simulink library "CryoDetLibCMB"  (R2016b)
settings: Solver=VariableStepAuto  StartTime=0.0  StopTime=10.0  RelTol=1e-3
undefined symbols (not defined in the file): Fclk, xlipgetpartsetting
libraries: xbsIndex_r4 x329, CryoDetLibCMB x20, CryoDetLib x2, simulink x1
(part 2 of 3)

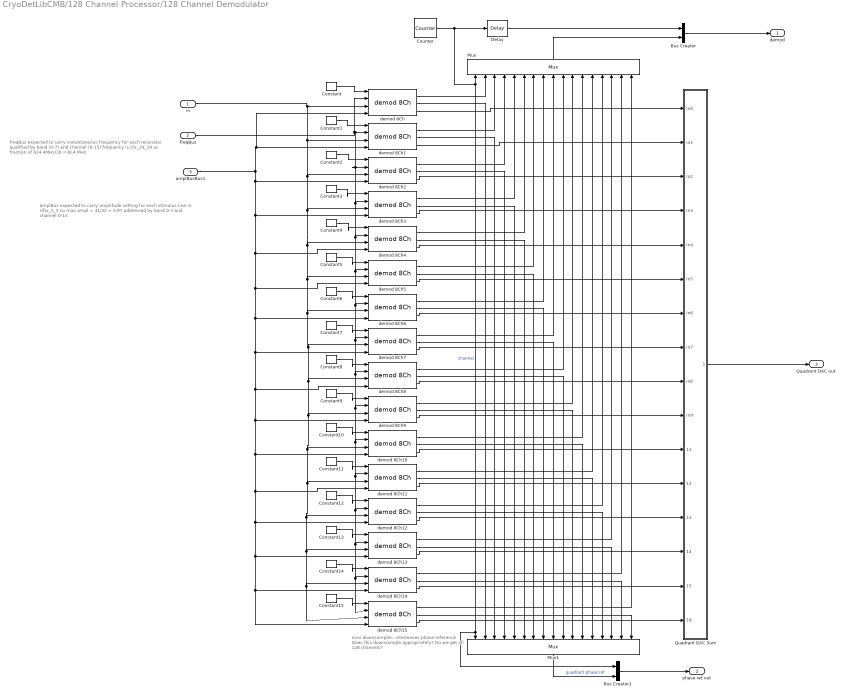
== system CryoDetLibCMB/128 Channel Processor/128 Channel Demodulator ==
  note: amplBus expected to carry  amplitude setting for each stimulus line
      | in Ufix_5_5 so max ampl = 31/32 = 0.97
      | addressed by band 0-7 and channel 0-15
  note: freqBus expected to carry instantaneous frequency for each resonator
      | qualified by band (0-7) and channel (0-15)
      | frequency is Fix_24_24 as fraction of 614.4MHz/16 =38.4 MHz
  note: mux downsamples, interleaves phase reference
      | Does this downsample appropriately?
      | Do we get all 128 channels?
  in : Inport
  freqBus : Inport  Port=2
  amplBusBus1 : Inport  Port=3
  Bus Creator : BusCreator  Inputs=2
  Bus Creator1 : BusCreator  Inputs=2
  Constant : xbsIndex_r4/Constant  const=0  gui_display_data_type=Fixed-point  arith_type=Unsigned  n_bits=4  bin_pt=0  preci_type=Single  exp_width=8  frac_width=24  explicit_period=off  period=1  equ=P=C  opselect=C  inp2=PCIN>>17  opr=+  inp1=P  carry=CIN  dbl_ovrd=off  block_type=constant
  Constant1 : xbsIndex_r4/Constant  const=1  gui_display_data_type=Fixed-point  arith_type=Unsigned  n_bits=4  bin_pt=0  preci_type=Single  exp_width=8  frac_width=24  explicit_period=off  period=1  equ=P=C  opselect=C  inp2=PCIN>>17  opr=+  inp1=P  carry=CIN  dbl_ovrd=off  block_type=constant
  Constant10 : xbsIndex_r4/Constant  const=10  gui_display_data_type=Fixed-point  arith_type=Unsigned  n_bits=4  bin_pt=0  preci_type=Single  exp_width=8  frac_width=24  explicit_period=off  period=1  equ=P=C  opselect=C  inp2=PCIN>>17  opr=+  inp1=P  carry=CIN  dbl_ovrd=off  block_type=constant
  Constant11 : xbsIndex_r4/Constant  const=11  gui_display_data_type=Fixed-point  arith_type=Unsigned  n_bits=4  bin_pt=0  preci_type=Single  exp_width=8  frac_width=24  explicit_period=off  period=1  equ=P=C  opselect=C  inp2=PCIN>>17  opr=+  inp1=P  carry=CIN  dbl_ovrd=off  block_type=constant
  Constant12 : xbsIndex_r4/Constant  const=12  gui_display_data_type=Fixed-point  arith_type=Unsigned  n_bits=4  bin_pt=0  preci_type=Single  exp_width=8  frac_width=24  explicit_period=off  period=1  equ=P=C  opselect=C  inp2=PCIN>>17  opr=+  inp1=P  carry=CIN  dbl_ovrd=off  block_type=constant
  Constant13 : xbsIndex_r4/Constant  const=13  gui_display_data_type=Fixed-point  arith_type=Unsigned  n_bits=4  bin_pt=0  preci_type=Single  exp_width=8  frac_width=24  explicit_period=off  period=1  equ=P=C  opselect=C  inp2=PCIN>>17  opr=+  inp1=P  carry=CIN  dbl_ovrd=off  block_type=constant
  Constant14 : xbsIndex_r4/Constant  const=14  gui_display_data_type=Fixed-point  arith_type=Unsigned  n_bits=4  bin_pt=0  preci_type=Single  exp_width=8  frac_width=24  explicit_period=off  period=1  equ=P=C  opselect=C  inp2=PCIN>>17  opr=+  inp1=P  carry=CIN  dbl_ovrd=off  block_type=constant
  Constant15 : xbsIndex_r4/Constant  const=15  gui_display_data_type=Fixed-point  arith_type=Unsigned  n_bits=4  bin_pt=0  preci_type=Single  exp_width=8  frac_width=24  explicit_period=off  period=1  equ=P=C  opselect=C  inp2=PCIN>>17  opr=+  inp1=P  carry=CIN  dbl_ovrd=off  block_type=constant
  Constant2 : xbsIndex_r4/Constant  const=2  gui_display_data_type=Fixed-point  arith_type=Unsigned  n_bits=4  bin_pt=0  preci_type=Single  exp_width=8  frac_width=24  explicit_period=off  period=1  equ=P=C  opselect=C  inp2=PCIN>>17  opr=+  inp1=P  carry=CIN  dbl_ovrd=off  block_type=constant
  Constant3 : xbsIndex_r4/Constant  const=3  gui_display_data_type=Fixed-point  arith_type=Unsigned  n_bits=4  bin_pt=0  preci_type=Single  exp_width=8  frac_width=24  explicit_period=off  period=1  equ=P=C  opselect=C  inp2=PCIN>>17  opr=+  inp1=P  carry=CIN  dbl_ovrd=off  block_type=constant
  Constant4 : xbsIndex_r4/Constant  const=4  gui_display_data_type=Fixed-point  arith_type=Unsigned  n_bits=4  bin_pt=0  preci_type=Single  exp_width=8  frac_width=24  explicit_period=off  period=1  equ=P=C  opselect=C  inp2=PCIN>>17  opr=+  inp1=P  carry=CIN  dbl_ovrd=off  block_type=constant
  Constant5 : xbsIndex_r4/Constant  const=5  gui_display_data_type=Fixed-point  arith_type=Unsigned  n_bits=4  bin_pt=0  preci_type=Single  exp_width=8  frac_width=24  explicit_period=off  period=1  equ=P=C  opselect=C  inp2=PCIN>>17  opr=+  inp1=P  carry=CIN  dbl_ovrd=off  block_type=constant
  Constant6 : xbsIndex_r4/Constant  const=6  gui_display_data_type=Fixed-point  arith_type=Unsigned  n_bits=4  bin_pt=0  preci_type=Single  exp_width=8  frac_width=24  explicit_period=off  period=1  equ=P=C  opselect=C  inp2=PCIN>>17  opr=+  inp1=P  carry=CIN  dbl_ovrd=off  block_type=constant
  Constant7 : xbsIndex_r4/Constant  const=7  gui_display_data_type=Fixed-point  arith_type=Unsigned  n_bits=4  bin_pt=0  preci_type=Single  exp_width=8  frac_width=24  explicit_period=off  period=1  equ=P=C  opselect=C  inp2=PCIN>>17  opr=+  inp1=P  carry=CIN  dbl_ovrd=off  block_type=constant
  Constant8 : xbsIndex_r4/Constant  const=8  gui_display_data_type=Fixed-point  arith_type=Unsigned  n_bits=4  bin_pt=0  preci_type=Single  exp_width=8  frac_width=24  explicit_period=off  period=1  equ=P=C  opselect=C  inp2=PCIN>>17  opr=+  inp1=P  carry=CIN  dbl_ovrd=off  block_type=constant
  Constant9 : xbsIndex_r4/Constant  const=9  gui_display_data_type=Fixed-point  arith_type=Unsigned  n_bits=4  bin_pt=0  preci_type=Single  exp_width=8  frac_width=24  explicit_period=off  period=1  equ=P=C  opselect=C  inp2=PCIN>>17  opr=+  inp1=P  carry=CIN  dbl_ovrd=off  block_type=constant
  Counter : xbsIndex_r4/Counter  cnt_type=Free Running  cnt_to=Inf  operation=Up  start_count=0  cnt_by_val=1  arith_type=Unsigned  n_bits=4  bin_pt=0  load_pin=off  rst=off  en=off  explicit_period=on  period=Tclk  use_behavioral_HDL=off  implementation=Fabric  dbl_ovrd=off  block_type=counter
  Delay : xbsIndex_r4/Delay  rst=off  infoeditControl=Selection of Reset will increase slice count due to use of real FFs and instead of SRLs  en=off  latency=1  reg_retiming=off  dbl_ovrd=off  block_type=delay
  Mux : xbsIndex_r4/Mux  inputs=16  en=off  latency=1  precision=Full  arith_type=Unsigned  n_bits=16  bin_pt=14  quantization=Truncate  overflow=Wrap  dbl_ovrd=off  block_type=mux
  Mux1 : xbsIndex_r4/Mux  inputs=16  en=off  latency=1  precision=Full  arith_type=Unsigned  n_bits=16  bin_pt=14  quantization=Truncate  overflow=Wrap  dbl_ovrd=off  block_type=mux
  Quadrant DAC Sum : Subsystem
  demod 8Ch{,1..15} (16 alike) : CryoDetLibCMB/demod 8Ch
  demod : Outport
  phase ref out : Outport  Port=2
  Quadrant DAC out : Outport  Port=3
  wires:
  Constant/1 -> demod 8Ch/1
  Constant1/1 -> demod 8Ch1/1
  Constant2/1 -> demod 8Ch2/1
  Constant3/1 -> demod 8Ch3/1
  Constant4/1 -> demod 8Ch4/1
  Constant5/1 -> demod 8Ch5/1
  Constant6/1 -> demod 8Ch6/1
  Constant7/1 -> demod 8Ch7/1
  Constant8/1 -> demod 8Ch8/1
  Constant9/1 -> demod 8Ch9/1
  Constant10/1 -> demod 8Ch10/1
  Constant11/1 -> demod 8Ch11/1
  Constant12/1 -> demod 8Ch12/1
  Constant13/1 -> demod 8Ch13/1
  Constant14/1 -> demod 8Ch14/1
  freqBus/1 -> demod 8Ch2/2, demod 8Ch5/2, demod 8Ch6/2, demod 8Ch7/2, demod 8Ch8/2, demod 8Ch10/2, demod 8Ch11/2, demod 8Ch12/2, demod 8Ch13/2, demod 8Ch14/2, demod 8Ch15/2, demod 8Ch9/2, demod 8Ch4/2, demod 8Ch3/2, demod 8Ch1/2, demod 8Ch/2
  demod 8Ch/1 -> Mux/2
  Counter/1 -> Delay/1, Bus Creator1/1, Mux1/1, Mux/1  "channel"
  Delay/1 -> Bus Creator/1
  Mux/1 -> Bus Creator/2
  demod 8Ch1/1 -> Mux/3
  demod 8Ch2/1 -> Mux/4
  demod 8Ch3/1 -> Mux/5
  demod 8Ch4/1 -> Mux/6
  demod 8Ch5/1 -> Mux/7
  demod 8Ch/2 -> Mux1/2
  demod 8Ch1/2 -> Mux1/3
  demod 8Ch2/2 -> Mux1/4
  demod 8Ch3/2 -> Mux1/5
  demod 8Ch4/2 -> Mux1/6
  demod 8Ch5/2 -> Mux1/7
  demod 8Ch/3 -> Quadrant DAC Sum/1(In0)
  demod 8Ch1/3 -> Quadrant DAC Sum/2(In1)
  demod 8Ch2/3 -> Quadrant DAC Sum/3(In2)
  demod 8Ch3/3 -> Quadrant DAC Sum/4(In3)
  demod 8Ch4/3 -> Quadrant DAC Sum/5(In4)
  demod 8Ch5/3 -> Quadrant DAC Sum/6(In5)
  demod 8Ch6/3 -> Quadrant DAC Sum/7(In6)
  demod 8Ch7/3 -> Quadrant DAC Sum/8(In7)
  demod 8Ch8/3 -> Quadrant DAC Sum/9(In8)
  demod 8Ch9/3 -> Quadrant DAC Sum/10(In9)
  demod 8Ch10/3 -> Quadrant DAC Sum/11(In10)
  demod 8Ch11/3 -> Quadrant DAC Sum/12(In11)
  demod 8Ch12/3 -> Quadrant DAC Sum/13(In12)
  demod 8Ch13/3 -> Quadrant DAC Sum/14(In13)
  demod 8Ch14/3 -> Quadrant DAC Sum/15(In14)
  Constant15/1 -> demod 8Ch15/1
  demod 8Ch15/3 -> Quadrant DAC Sum/16(In15)
  demod 8Ch15/2 -> Mux1/17
  demod 8Ch14/2 -> Mux1/16
  demod 8Ch13/2 -> Mux1/15
  demod 8Ch6/1 -> Mux/8
  demod 8Ch7/1 -> Mux/9
  demod 8Ch8/1 -> Mux/10
  demod 8Ch9/1 -> Mux/11
  demod 8Ch10/1 -> Mux/12
  demod 8Ch11/1 -> Mux/13
  demod 8Ch12/1 -> Mux/14
  demod 8Ch13/1 -> Mux/15
  demod 8Ch14/1 -> Mux/16
  demod 8Ch15/1 -> Mux/17
  demod 8Ch6/2 -> Mux1/8
  demod 8Ch12/2 -> Mux1/14
  demod 8Ch11/2 -> Mux1/13
  demod 8Ch10/2 -> Mux1/12
  demod 8Ch9/2 -> Mux1/11
  demod 8Ch7/2 -> Mux1/9
  demod 8Ch8/2 -> Mux1/10
  Mux1/1 -> Bus Creator1/2  "quadrant phase ref"
  Bus Creator1/1 -> phase ref out/1
  in/1 -> demod 8Ch/3, demod 8Ch2/3, demod 8Ch6/3, demod 8Ch7/3, demod 8Ch8/3, demod 8Ch10/3, demod 8Ch12/3, demod 8Ch15/3, demod 8Ch14/3, demod 8Ch13/3, demod 8Ch11/3, demod 8Ch9/3, demod 8Ch5/3, demod 8Ch4/3, demod 8Ch3/3, demod 8Ch1/3
  Bus Creator/1 -> demod/1
  Quadrant DAC Sum/1(Out2) -> Quadrant DAC out/1
  amplBusBus1/1 -> demod 8Ch/4, demod 8Ch1/4, demod 8Ch4/4, demod 8Ch5/4, demod 8Ch6/4, demod 8Ch7/4, demod 8Ch8/4, demod 8Ch9/4, demod 8Ch10/4, demod 8Ch11/4, demod 8Ch12/4, demod 8Ch13/4, demod 8Ch14/4, demod 8Ch15/4, demod 8Ch3/4, demod 8Ch2/4

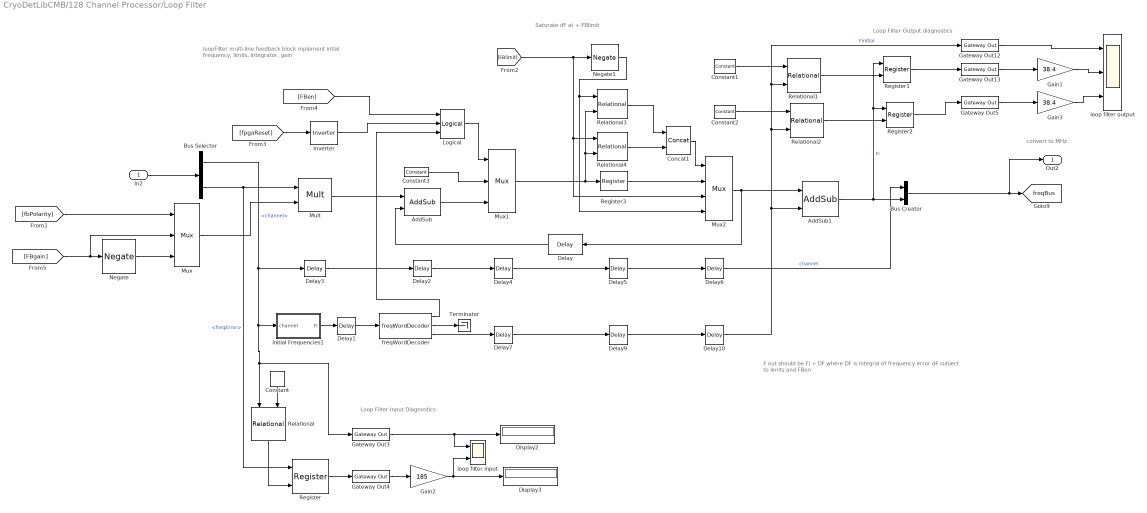
== system CryoDetLibCMB/128 Channel Processor/Loop Filter ==
  note: Loop Filter Output diagnostics
  note: Loop Filter Input Diagnostics
  note: Saturate dF at +-FBlimit
  note: convert to MHz
  note: F out should be Fi + DF
      | where DF is integral of frequency error dF subject to limits and FBen
  note: loopFilter
      | multi-line feedback block
      | mplement intial frequency, limits, integrator, gain
  In2 : Inport
  AddSub : xbsIndex_r4/AddSub  mode=Addition  use_carryin=off  use_carryout=off  en=off  latency=1  precision=User Defined  arith_type="Signed  (2's comp)"  n_bits=32  bin_pt=30  quantization=Truncate  overflow=Saturate  use_behavioral_HDL=off  hw_selection=Fabric  pipelined=off  dbl_ovrd=off  block_type=addsub
  AddSub1 : xbsIndex_r4/AddSub  mode=Addition  use_carryin=off  use_carryout=off  en=off  latency=1  precision=Full  arith_type=Unsigned  n_bits=16  bin_pt=14  quantization=Truncate  overflow=Wrap  use_behavioral_HDL=off  hw_selection=Fabric  pipelined=off  dbl_ovrd=off  block_type=addsub
  Bus Selector : BusSelector  OutputSignals=channel,freqError
  Bus Creator : BusCreator  Inputs=2
  Concat1 : xbsIndex_r4/Concat  num_inputs=2  dbl_ovrd=off  block_type=concat
  Constant : xbsIndex_r4/Constant  const=0  gui_display_data_type=Fixed-point  arith_type=Unsigned  n_bits=4  bin_pt=0  preci_type=Single  exp_width=8  frac_width=24  explicit_period=off  period=1  equ=P=C  opselect=C  inp2=PCIN>>17  opr=+  inp1=P  carry=CIN  dbl_ovrd=off  block_type=constant
  Constant1 : xbsIndex_r4/Constant  const=0  gui_display_data_type=Fixed-point  arith_type=Unsigned  n_bits=4  bin_pt=0  preci_type=Single  exp_width=8  frac_width=24  explicit_period=off  period=1  equ=P=C  opselect=C  inp2=PCIN>>17  opr=+  inp1=P  carry=CIN  dbl_ovrd=off  block_type=constant
  Constant2 : xbsIndex_r4/Constant  const=6  gui_display_data_type=Fixed-point  arith_type=Unsigned  n_bits=4  bin_pt=0  preci_type=Single  exp_width=8  frac_width=24  explicit_period=off  period=1  equ=P=C  opselect=C  inp2=PCIN>>17  opr=+  inp1=P  carry=CIN  dbl_ovrd=off  block_type=constant
  Constant3 : xbsIndex_r4/Constant  const=0  gui_display_data_type=Fixed-point  arith_type=Signed (2's comp)  n_bits=32  bin_pt=30  preci_type=Single  exp_width=8  frac_width=24  explicit_period=off  period=1  equ=P=C  opselect=C  inp2=PCIN>>17  opr=+  inp1=P  carry=CIN  dbl_ovrd=off  block_type=constant
  Delay : xbsIndex_r4/Delay  rst=off  infoeditControl=Selection of Reset will increase slice count due to use of real FFs and instead of SRLs  en=off  latency=124  reg_retiming=off  dbl_ovrd=off  block_type=delay
  Delay1 : xbsIndex_r4/Delay  rst=off  infoeditControl=Selection of Reset will increase slice count due to use of real FFs and instead of SRLs  en=off  latency=2  reg_retiming=off  dbl_ovrd=off  block_type=delay
  Delay{2,4..6,9..10} (6 alike) : xbsIndex_r4/Delay  rst=off  infoeditControl=Selection of Reset will increase slice count due to use of real FFs and instead of SRLs  en=off  latency=1  reg_retiming=off  dbl_ovrd=off  block_type=delay
  Delay3 : xbsIndex_r4/Delay  rst=off  infoeditControl=Selection of Reset will increase slice count due to use of real FFs and instead of SRLs  en=off  latency=3  reg_retiming=off  dbl_ovrd=off  block_type=delay
  Delay7 : xbsIndex_r4/Delay  rst=off  infoeditControl=Selection of Reset will increase slice count due to use of real FFs and instead of SRLs  en=off  latency=2  reg_retiming=off  dbl_ovrd=off  block_type=delay
  Display2 : Display
  Display3 : Display
  Gain1 : Gain  Gain=38.4
  Gain2 : Gain  Gain=185
  Gain3 : Gain  Gain=38.4
  Gateway Out12 : xbsIndex_r4/Gateway Out  inherit_from_input=off  hdl_port=off  rows=1  columns=1  UseAsDAC=off  DACChannel='1'  interface=None  automatic_assignment=on  address_offset=hex2dec('00')  intf_name=''  intf_description=''  timing_constraint=None  locs_specified=off  LOCs={}  io_standard={}  block_type=gatewayout
  Gateway Out13 : xbsIndex_r4/Gateway Out  inherit_from_input=on  hdl_port=off  rows=1  columns=1  UseAsDAC=off  DACChannel='1'  interface=None  automatic_assignment=on  address_offset=hex2dec('00')  intf_name=''  intf_description=''  timing_constraint=None  locs_specified=off  LOCs={}  io_standard={}  block_type=gatewayout
  Gateway Out3 : xbsIndex_r4/Gateway Out  inherit_from_input=off  hdl_port=off  rows=1  columns=1  UseAsDAC=off  DACChannel='1'  interface=None  automatic_assignment=on  address_offset=hex2dec('00')  intf_name=''  intf_description=''  timing_constraint=None  locs_specified=off  LOCs={}  io_standard={}  block_type=gatewayout
  Gateway Out4 : xbsIndex_r4/Gateway Out  inherit_from_input=off  hdl_port=off  rows=1  columns=1  UseAsDAC=off  DACChannel='1'  interface=None  automatic_assignment=on  address_offset=hex2dec('00')  intf_name=''  intf_description=''  timing_constraint=None  locs_specified=off  LOCs={}  io_standard={}  block_type=gatewayout
  Gateway Out5 : xbsIndex_r4/Gateway Out  inherit_from_input=on  hdl_port=off  rows=1  columns=1  UseAsDAC=off  DACChannel='1'  interface=None  automatic_assignment=on  address_offset=hex2dec('00')  intf_name=''  intf_description=''  timing_constraint=None  locs_specified=off  LOCs={}  io_standard={}  block_type=gatewayout
  Inverter : xbsIndex_r4/Inverter  en=off  latency=1  dbl_ovrd=off  block_type=inv
  Logical : xbsIndex_r4/Logical  logical_function=OR  inputs=3  en=off  latency=1  precision=User Defined  arith_type=Boolean  n_bits=16  bin_pt=0  align_bp=on  dbl_ovrd=off  block_type=logical
  Mult : xbsIndex_r4/Mult  precision=User Defined  arith_type="Signed  (2's comp)"  n_bits=32  bin_pt=30  quantization=Truncate  overflow=Saturate  en=off  latency=3  use_behavioral_HDL=off  opt=Speed  use_embedded=on  optimum_pipeline=off  pipeline=on  dbl_ovrd=off  use_rpm=on  placement_style=Triangular  block_type=mult
  Mux : xbsIndex_r4/Mux  inputs=2  en=off  latency=1  precision=Full  arith_type=Unsigned  n_bits=16  bin_pt=14  quantization=Truncate  overflow=Wrap  dbl_ovrd=off  block_type=mux
  Mux1 : xbsIndex_r4/Mux  inputs=2  en=off  latency=1  precision=Full  arith_type=Unsigned  n_bits=16  bin_pt=14  quantization=Truncate  overflow=Wrap  dbl_ovrd=off  block_type=mux
  Mux2 : xbsIndex_r4/Mux  inputs=3  en=off  latency=1  precision=Full  arith_type=Unsigned  n_bits=16  bin_pt=14  quantization=Truncate  overflow=Wrap  dbl_ovrd=off  block_type=mux
  Negate : xbsIndex_r4/Negate  precision=Full  arith_type=Unsigned  n_bits=16  bin_pt=14  quantization=Truncate  overflow=Wrap  en=off  latency=1  dbl_ovrd=off  block_type=negate
  Negate1 : xbsIndex_r4/Negate  precision=Full  arith_type=Unsigned  n_bits=16  bin_pt=14  quantization=Truncate  overflow=Wrap  en=off  latency=1  dbl_ovrd=off  block_type=negate
  Register : xbsIndex_r4/Register  init=0  rst=off  en=on  dbl_ovrd=off  block_type=register
  Register1 : xbsIndex_r4/Register  init=0  rst=off  en=on  dbl_ovrd=off  block_type=register
  Register2 : xbsIndex_r4/Register  init=0  rst=off  en=on  dbl_ovrd=off  block_type=register
  Register3 : xbsIndex_r4/Register  init=0  rst=off  en=off  dbl_ovrd=off  block_type=register
  Relational : xbsIndex_r4/Relational  mode=a=b  op_type=Bool  en=off  latency=0  dbl_ovrd=off  block_type=relational
  Relational1 : xbsIndex_r4/Relational  mode=a=b  op_type=Bool  en=off  latency=0  dbl_ovrd=off  block_type=relational
  Relational2 : xbsIndex_r4/Relational  mode=a=b  op_type=Bool  en=off  latency=0  dbl_ovrd=off  block_type=relational
  Relational3 : xbsIndex_r4/Relational  mode=a>b  op_type=Bool  en=off  latency=1  dbl_ovrd=off  block_type=relational
  Relational4 : xbsIndex_r4/Relational  mode=a<b  op_type=Bool  en=off  latency=1  dbl_ovrd=off  block_type=relational
  Terminator : Terminator
  freqWordDecoder : CryoDetLibCMB/freqWordDecoder
  initial Frequencies1 : Subsystem
  loop filter input : Scope  NumInputPorts=2
  loop filter output : Scope  NumInputPorts=3
  Out2 : Outport
  tag scope: freqBus=global
  wires:
  In2/1 -> Bus Selector/1
  Bus Selector/1 -> initial Frequencies1/1(channel), Relational/1, Gateway Out3/1, Delay3/1  "<channel>"
  Bus Selector/2 -> Mult/1, Register/1  "<freqError>"
  Bus Creator/1 -> Out2/1, [freqBus]
  [fbPolarity] -> Mux/1
  [FBgain] -> Mux/2, Negate/1
  [FBlimit] -> Negate1/1, Mux2/3, Relational4/1
  initial Frequencies1/1(Fi) -> Delay1/1
  Gateway Out13/1 -> Gain1/1
  Gateway Out12/1 -> loop filter output/1
  Gateway Out4/1 -> Gain2/1
  Gateway Out3/1 -> loop filter input/1, Display2/1
  Constant/1 -> Relational/2
  Relational/1 -> Register/2
  Register/1 -> Gateway Out4/1
  Constant1/1 -> Relational1/1
  Relational1/1 -> Register1/2
  Register1/1 -> Gateway Out13/1
  Gain1/1 -> loop filter output/2
  Gain2/1 -> Display3/1, loop filter input/2
  Constant2/1 -> Relational2/1
  Relational2/1 -> Register2/2
  Register2/1 -> Gateway Out5/1
  Gateway Out5/1 -> Gain3/1
  Gain3/1 -> loop filter output/3
  Negate/1 -> Mux/3
  Mult/1 -> AddSub/1
  Mux/1 -> Mult/2
  [fpgaReset] -> Inverter/1
  [FBen] -> Logical/1
  Logical/1 -> Mux1/1
  AddSub/1 -> Mux1/3
  Constant3/1 -> Mux1/2
  Inverter/1 -> Logical/2
  Mux1/1 -> Register3/1, Relational4/2, Relational3/2
  Relational3/1 -> Concat1/1
  Relational4/1 -> Concat1/2
  Concat1/1 -> Mux2/1
  Negate1/1 -> Mux2/4, Relational3/1
  Register3/1 -> Mux2/2
  Delay/1 -> AddSub/2
  Mux2/1 -> AddSub1/1, Delay/1
  freqWordDecoder/2 -> Terminator/1
  freqWordDecoder/1 -> Logical/3
  Delay3/1 -> Delay2/1
  Delay2/1 -> Delay4/1
  Delay4/1 -> Delay5/1
  Delay5/1 -> Delay6/1
  freqWordDecoder/3 -> Delay7/1
  Delay1/1 -> freqWordDecoder/1
  Delay7/1 -> Delay9/1
  Delay9/1 -> Delay10/1
  Delay10/1 -> Relational2/2, Gateway Out12/1, Relational1/2, AddSub1/2  "Finitial"
  AddSub1/1 -> Register2/1, Register1/1, Bus Creator/2  "Fi"
  Delay6/1 -> Bus Creator/1  "channel"

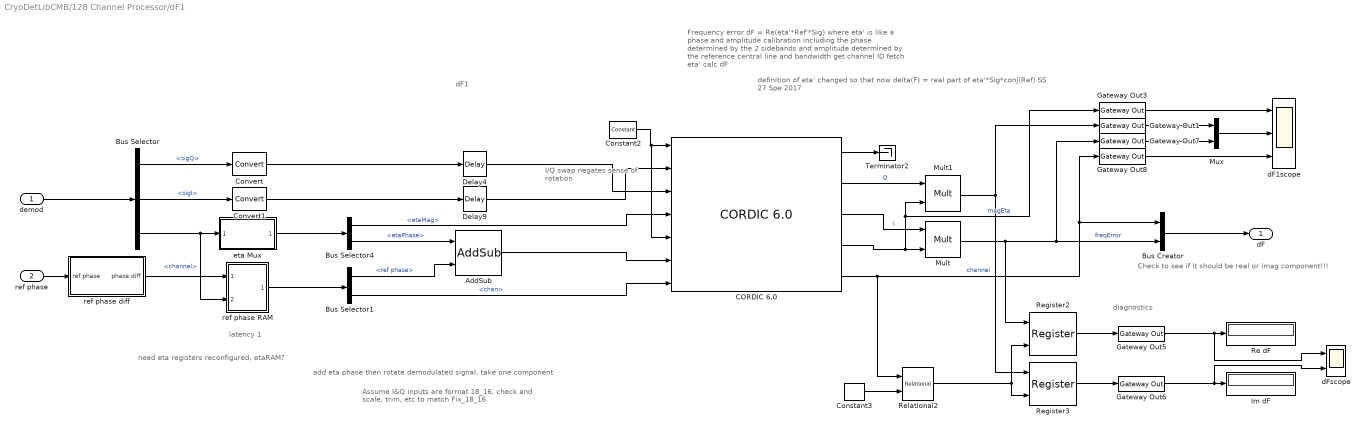
== system CryoDetLibCMB/128 Channel Processor/dF1 ==
  note: Check to see if it should be real or imag component!!!
  note: latency 1
  note: Assume I&Q inputs are format 18_16,
      | check and scale, trim, etc to match Fix_18_16
  note: I/Q swap negates sense of rotation
  note: need eta registers reconfigured, etaRAM?
  note: add eta phase then rotate demodulated signal, take one component
  note: definition of eta' changed so that now delta(F) = real part of eta'*Sig*conj(Ref)
      | SS 27 Spe 2017
  note: diagnostics
  note: dF1
  note: Frequency error dF = Re(eta'*Ref'*Sig)
      | where eta' is like a phase and amplitude calibration including the phase determined by the 2 sidebands and amplitude determined by the reference central line and bandwidth
      |
      | get channel ID
      | fetch eta'
      | calc dF
  demod : Inport
  ref phase : Inport  Port=2
  AddSub : xbsIndex_r4/AddSub  mode=Addition  use_carryin=off  use_carryout=off  en=off  latency=3  precision=User Defined  arith_type=Unsigned  n_bits=18  bin_pt=15  quantization=Truncate  overflow=Wrap  use_behavioral_HDL=off  hw_selection=Fabric  pipelined=off  dbl_ovrd=off  block_type=addsub
  Bus Selector : BusSelector  OutputSignals=SignalQ&I.sigQ,SignalQ&I.sigI,channel
  Bus Selector1 : BusSelector  OutputSignals=ref phase,chan
  Bus Selector4 : BusSelector  OutputSignals=etaMag,etaPhase
  Bus Creator : BusCreator  Inputs=2
  "CORDIC 6.0 " : xbsIndex_r4/CORDIC 6.0   functional_selection=Rotate  architectural_configuration=Parallel  pipelining_mode=Optimal  data_format=SignedFraction  phase_format=Scaled_Radians  input_width=17  output_width=18  round_mode=Truncate  iterations=0  precision=0  compensation_scaling=No_Scale_Compensation  coarse_rotation=on  aclken=off  aresetn=off  out_tready=off  cartesian_has_tuser=on  cartesian_has_tlast=off  cartesian_tuser_width=16  phase_has_tuser=on  phase_has_tlast=off  phase_tuser_width=4  out_tlast_behv=Null  flow_control=NonBlocking  optimize_goal=Resources  trim_axipin_name=on  simulation_type=hybrid_sim  simulation_model=sysgen:cordic_v6_0  data_path_portlist={'s_axis_cartesian_tdata_imag', 's_axis_cartesian_tdata_real', 's_axis_phase_tdata_phase', 'm_axis_dout_tdata_imag', 'm_axis_dout_tdata_real', 'm_axis_dout_tdata_phase','m_axis_dout_tdata'}  ip_name=CORDIC  ip_version=6.0  dsptool_ready=true  ipcore_usecache=true  ipcore_useipmodelcache=true  wrapper_available=true  port_translation_map={ 'aclken' => 'en', 'aresetn' => 'rst' }  block_type=cordic_v6_0
      settings: infoedit=CORDIC 6.0
  Constant2 : xbsIndex_r4/Constant  const=1  gui_display_data_type=Boolean  arith_type=Boolean  n_bits=16  bin_pt=14  preci_type=Single  exp_width=8  frac_width=24  explicit_period=off  period=1  equ=P=C  opselect=C  inp2=PCIN>>17  opr=+  inp1=P  carry=CIN  dbl_ovrd=off  block_type=constant
  Constant3 : xbsIndex_r4/Constant  const=0  gui_display_data_type=Fixed-point  arith_type=Unsigned  n_bits=4  bin_pt=0  preci_type=Single  exp_width=8  frac_width=24  explicit_period=off  period=1  equ=P=C  opselect=C  inp2=PCIN>>17  opr=+  inp1=P  carry=CIN  dbl_ovrd=off  block_type=constant
  Convert : xbsIndex_r4/Convert  gui_display_data_type=Fixed-point  arith_type="Signed  (2's comp)"  n_bits=18  bin_pt=16  float_type=Single  exp_bits=8  fraction_bits=24  quantization=Truncate  overflow=Saturate  en=off  latency=1  pipeline=off  dbl_ovrd=off  block_type=convert
  Convert1 : xbsIndex_r4/Convert  gui_display_data_type=Fixed-point  arith_type="Signed  (2's comp)"  n_bits=18  bin_pt=16  float_type=Single  exp_bits=8  fraction_bits=24  quantization=Truncate  overflow=Saturate  en=off  latency=1  pipeline=off  dbl_ovrd=off  block_type=convert
  Delay4 : xbsIndex_r4/Delay  rst=off  infoeditControl=Selection of Reset will increase slice count due to use of real FFs and instead of SRLs  en=off  latency=3  reg_retiming=on  dbl_ovrd=off  block_type=delay
  Delay9 : xbsIndex_r4/Delay  rst=off  infoeditControl=Selection of Reset will increase slice count due to use of real FFs and instead of SRLs  en=off  latency=3  reg_retiming=on  dbl_ovrd=off  block_type=delay
  Gateway Out{1,3,5..8} (6 alike) : xbsIndex_r4/Gateway Out  inherit_from_input=off  hdl_port=off  rows=1  columns=1  UseAsDAC=off  DACChannel='1'  interface=None  automatic_assignment=on  address_offset=hex2dec('00')  intf_name=''  intf_description=''  timing_constraint=None  locs_specified=off  LOCs={}  io_standard={}  block_type=gatewayout
  Im dF : Display
  Mult : xbsIndex_r4/Mult  precision=Full  arith_type="Signed  (2's comp)"  n_bits=16  bin_pt=14  quantization=Truncate  overflow=Wrap  en=off  latency=3  use_behavioral_HDL=off  opt=Speed  use_embedded=on  optimum_pipeline=off  pipeline=on  dbl_ovrd=off  use_rpm=on  placement_style=Triangular  block_type=mult
  Mult1 : xbsIndex_r4/Mult  precision=Full  arith_type="Signed  (2's comp)"  n_bits=16  bin_pt=14  quantization=Truncate  overflow=Wrap  en=off  latency=3  use_behavioral_HDL=off  opt=Speed  use_embedded=on  optimum_pipeline=off  pipeline=on  dbl_ovrd=off  use_rpm=on  placement_style=Triangular  block_type=mult
  Mux : Mux  Inputs=2
  Re dF : Display
  Register2 : xbsIndex_r4/Register  init=0  rst=off  en=on  dbl_ovrd=off  block_type=register
  Register3 : xbsIndex_r4/Register  init=0  rst=off  en=on  dbl_ovrd=off  block_type=register
  Relational2 : xbsIndex_r4/Relational  mode=a=b  op_type=Bool  en=off  latency=0  dbl_ovrd=off  block_type=relational
  Terminator2 : Terminator
  "dF1scope " : Scope  NumInputPorts=3
  dFscope : Scope  NumInputPorts=2
  eta Mux : Subsystem
  ref phase RAM : Subsystem
  ref phase diff : Subsystem
  dF : Outport
  wires:
  demod/1 -> Bus Selector/1
  Bus Selector/3 -> eta Mux/1(channel), ref phase RAM/2(read channel)  "<channel>"
  eta Mux/1(eta out) -> Bus Selector4/1
  Constant3/1 -> Relational2/2
  Relational2/1 -> Register3/2, Register2/2
  Register2/1 -> Gateway Out5/1
  Gateway Out5/1 -> dFscope/1, Re dF/1
  Gateway Out6/1 -> dFscope/2, Im dF/1
  Register3/1 -> Gateway Out6/1
  "CORDIC 6.0 "/1 -> Terminator2/1
  Gateway Out3/1 -> "dF1scope "/1
  ref phase/1 -> ref phase diff/1(ref phase)
  ref phase diff/1(phase diff) -> ref phase RAM/1(ref Phase)
  AddSub/1 -> "CORDIC 6.0 "/6
  Bus Selector/1 -> Convert/1  "<sigQ>"
  Bus Selector4/2 -> AddSub/1  "<etaPhase>"
  ref phase RAM/1(ref phase) -> Bus Selector1/1
  Bus Selector1/1 -> AddSub/2  "<ref phase>"
  Bus Selector1/2 -> "CORDIC 6.0 "/7  "<chan>"
  Delay4/1 -> "CORDIC 6.0 "/3
  Delay9/1 -> "CORDIC 6.0 "/2
  Bus Selector4/1 -> "CORDIC 6.0 "/4  "<etaMag>"
  Constant2/1 -> "CORDIC 6.0 "/5, "CORDIC 6.0 "/1
  "CORDIC 6.0 "/4 -> Mult1/2, Gateway Out3/1, Mult/2  "magEta"
  "CORDIC 6.0 "/3 -> Mult/1  "I"
  "CORDIC 6.0 "/2 -> Mult1/1  "Q"
  Convert/1 -> Delay4/1
  Convert1/1 -> Delay9/1
  Bus Selector/2 -> Convert1/1  "<sigI>"
  Mux/1 -> "dF1scope "/2
  Gateway Out1/1 -> Mux/1
  Gateway Out7/1 -> Mux/2
  Gateway Out8/1 -> "dF1scope "/3
  Mult1/1 -> Register3/1, Gateway Out1/1
  Mult/1 -> Register2/1, Gateway Out7/1, Bus Creator/2  "freqError"
  "CORDIC 6.0 "/5 -> Relational2/1, Gateway Out8/1, Bus Creator/1  "channel"
  Bus Creator/1 -> dF/1

== system CryoDetLibCMB/demod 8Ch/CIC reset ==
  note: where N is number of channels in CIC filter
  note: reset latched resetIn
  note: latch resetIn
  note: CIC reset
      |
      | Synchronizes a CIC compiler 4.0 multi-channel CIC filter
      | to input channels
      |
      | Generates:
      | 1	notResetOut to CIC aresetn
      | 2	tlast to CIC tlast input
      |
      | Inputs:
      | 1	reset in
      | 2	Channel number (0-N) which may go to sel input of mux generating the input data stream
      | 3	N-2 which tells this module how deep is the multiplexing (e.g. N-2 = 10 for a 12 channel CIC filter (sorry))
      |
      | Guarantees:
      | 1	reset out is at least 2 clocks long
      | 2	end of reset occurs 2 clocks before channel 0
      | 3	tlast comes with channel N-1
      |
      | Assumes:
      | CIC oversampling set to "Sample period" = 1
      | No "streaming interface"
  resetIn : Inport
  Channel : Inport  Port=2
  N-2 : Inport  Port=3
  Constant : xbsIndex_r4/Constant  const=0  gui_display_data_type=Boolean  arith_type=Boolean  n_bits=16  bin_pt=14  preci_type=Single  exp_width=8  frac_width=24  explicit_period=off  period=1  equ=P=C  opselect=C  inp2=PCIN>>17  opr=+  inp1=P  carry=CIN  dbl_ovrd=off  block_type=constant
  Delay1 : xbsIndex_r4/Delay  rst=off  infoeditControl=Selection of Reset will increase slice count due to use of real FFs and instead of SRLs  en=off  latency=1  reg_retiming=off  dbl_ovrd=off  block_type=delay
  Delay2 : xbsIndex_r4/Delay  rst=off  infoeditControl=Selection of Reset will increase slice count due to use of real FFs and instead of SRLs  en=off  latency=1  reg_retiming=off  dbl_ovrd=off  block_type=delay
  Delay3 : xbsIndex_r4/Delay  rst=off  infoeditControl=Selection of Reset will increase slice count due to use of real FFs and instead of SRLs  en=off  latency=1  reg_retiming=off  dbl_ovrd=off  block_type=delay
  Inverter : xbsIndex_r4/Inverter  en=off  latency=2  dbl_ovrd=off  block_type=inv
  Inverter1 : xbsIndex_r4/Inverter  en=off  latency=0  dbl_ovrd=off  block_type=inv
  Logical : xbsIndex_r4/Logical  logical_function=AND  inputs=4  en=off  latency=0  precision=User Defined  arith_type=Boolean  n_bits=1  bin_pt=0  align_bp=on  dbl_ovrd=off  block_type=logical
  Logical1 : xbsIndex_r4/Logical  logical_function=OR  inputs=2  en=off  latency=0  precision=User Defined  arith_type=Boolean  n_bits=1  bin_pt=0  align_bp=on  dbl_ovrd=off  block_type=logical
  Mux : xbsIndex_r4/Mux  inputs=2  en=off  latency=0  precision=Full  arith_type=Unsigned  n_bits=16  bin_pt=14  quantization=Truncate  overflow=Wrap  dbl_ovrd=off  block_type=mux
  Relational1 : xbsIndex_r4/Relational  mode=a=b  op_type=Bool  en=off  latency=0  dbl_ovrd=off  block_type=relational
  notResetOut : Outport
  tlast : Outport  Port=2
  wires:
  resetIn/1 -> Inverter/1, Logical1/1
  Channel/1 -> Relational1/1
  N-2/1 -> Relational1/2
  Relational1/1 -> Logical/4, Delay1/1
  Logical1/1 -> Inverter1/1, Delay2/1
  Mux/1 -> Logical1/2
  Delay2/1 -> Logical/2, Delay3/1, Mux/2
  Constant/1 -> Mux/3
  Logical/1 -> Mux/1
  Delay1/1 -> tlast/1
  Inverter/1 -> Logical/1
  Delay3/1 -> Logical/3
  Inverter1/1 -> notResetOut/1

== system CryoDetLibCMB/demod 8Ch/DDS 8ch ==
  note: 8 Channel DDS
      | Given its channel ID, takes instantaneous frequency for this channel of each band and generates phase and I&Q
      | interleaved over 8 bands
      | Frequency RAM is updated asynchronously to operation
  note: Phase Accumulator
      | (8 Channels)
  note: Frequency RAM
  note: Sinc/Cos Generator
  note: Which demodulator channel is this?
  ID : Inport
  freqBus : Inport  Port=2
  band : Inport  Port=3
  AddSub : xbsIndex_r4/AddSub  mode=Addition  use_carryin=off  use_carryout=off  en=off  latency=3  precision=User Defined  arith_type=Unsigned  n_bits=24  bin_pt=24  quantization=Truncate  overflow=Wrap  use_behavioral_HDL=off  hw_selection=Fabric  pipelined=off  dbl_ovrd=off  block_type=addsub
  Bus Creator : BusCreator  Inputs=3
  Bus Creator1 : BusCreator  Inputs=2
  Bus Selector : BusSelector  OutputSignals=subBand,chan,freq
  Constant : xbsIndex_r4/Constant  const=1.0  gui_display_data_type=Boolean  arith_type=Boolean  n_bits=16  bin_pt=14  preci_type=Single  exp_width=8  frac_width=24  explicit_period=off  period=1  equ=P=C  opselect=C  inp2=PCIN>>17  opr=+  inp1=P  carry=CIN  dbl_ovrd=off  block_type=constant
  Convert : xbsIndex_r4/Convert  gui_display_data_type=Fixed-point  arith_type=Unsigned  n_bits=16  bin_pt=16  float_type=Single  exp_bits=8  fraction_bits=24  quantization=Truncate  overflow=Wrap  en=off  latency=1  pipeline=off  dbl_ovrd=off  block_type=convert
  "DDS Compiler 6.0 " : xbsIndex_r4/DDS Compiler 6.0   partspresent=SIN_COS_LUT_only  dds_clock_rate=100  channels=1  mode_of_operation=Standard  modulus=9  parameter_entry=System_Parameters  spurious_free_dynamic_range=45  frequency_resolution=0.4  noise_shaping=None  phase_width=16  output_width=16  output_selection=Sine_and_Cosine  negative_sine=off  negative_cosine=off  amplitude_mode=Full_Range  memory_type=Auto  optimization_goal=Auto  dsp48_use=Minimal  resync=off  latency_configuration=Auto  latency=1  has_phase_out=off  has_aclken=off  has_aresetn=off  explicit_period=off  period=1  data_has_tlast=Not_Required  has_tready=off  s_phase_has_tuser=User_Field  m_data_has_tuser=User_Field  m_phase_has_tuser=Not_Required  s_phase_tuser_width=3  output_form=Twos_Complement  s_config_sync_mode=On_Vector  phase_increment=Streaming  output_frequency1=0  output_frequency2=0  output_frequency3=0  output_frequency4=0  output_frequency5=0  output_frequency6=0  output_frequency7=0  output_frequency8=0  output_frequency9=0  output_frequency10=0  output_frequency11=0  output_frequency12=0  output_frequency13=0  output_frequency14=0  output_frequency15=0  output_frequency16=0  pinc1='0'  pinc2='0'  pinc3='0'  pinc4='0'  pinc5='0'  pinc6='0'  pinc7='0'  pinc8='0'  pinc9='0'  pinc10='0'  pinc11='0'  pinc12='0'  pinc13='0'  pinc14='0'  pinc15='0'  pinc16='0'  phase_offset=Streaming  phase_offset_angles1=0  phase_offset_angles2=0  phase_offset_angles3=0  phase_offset_angles4=0  phase_offset_angles5=0  phase_offset_angles6=0  phase_offset_angles7=0  phase_offset_angles8=0  phase_offset_angles9=0  phase_offset_angles10=0  phase_offset_angles11=0  phase_offset_angles12=0  phase_offset_angles13=0  phase_offset_angles14=0  phase_offset_angles15=0  phase_offset_angles16=0  poff1='0'  poff2='0'  poff3='0'  poff4='0'  poff5='0'  poff6='0'  poff7='0'  poff8='0'  poff9='0'  poff10='0'  poff11='0'  poff12='0'  poff13='0'  poff14='0'  poff15='0'  poff16='0'  trim_axipin_name=on  simulation_type=hybrid_sim  simulation_model=sysgen:xddsv6_0_cmodel  data_path_portlist={ 's_axis_config_tdata_poff', 's_axis_config_tdata_chan0_poff', 's_axis_config_tdata_pinc', 's_axis_config_tdata_chan0_pinc', 's_axis_phase_tdata_resync', 's_axis_phase_tdata_chan0_resync', 's_axis_phase_tdata_poff', 's_axis_phase_tdata_chan0_poff', 's_axis_phase_tdata_pinc', 's_axis_phase_tdata_chan0_pinc', 's_axis_phase_tdata_phase_in', 'm_axis_data_tdata_sine', 'm_axis_data_tdata_chan0_sine', 'm_axis_data_tdata_cosine', 'm_axis_data_tdata_chan0_cosine', 'm_axis_phase_tdata_phase_out', 'm_axis_phase_tdata_chan0_phase_out'}  por_mode=false  gui_behaviour=Sysgen  ip_name=DDS Compiler  ip_version=6.0  dsptool_ready=true  wrapper_available=true  port_translation_map={ 'aclken' => 'en', 'aresetn' => 'rst' }  ipcore_usecache=true  ipcore_useipmodelcache=true  ipcore_xco_need_fpga_part=true  ipcore_verbose=false  block_type=dds_compiler_v6_0
  Delay : xbsIndex_r4/Delay  rst=off  infoeditControl=Selection of Reset will increase slice count due to use of real FFs and instead of SRLs  en=off  latency=5  reg_retiming=off  dbl_ovrd=off  block_type=delay
  Delay1 : xbsIndex_r4/Delay  rst=off  infoeditControl=Selection of Reset will increase slice count due to use of real FFs and instead of SRLs  en=off  latency=3  reg_retiming=off  dbl_ovrd=off  block_type=delay
  Delay2 : xbsIndex_r4/Delay  rst=off  infoeditControl=Selection of Reset will increase slice count due to use of real FFs and instead of SRLs  en=off  latency=1  reg_retiming=off  dbl_ovrd=off  block_type=delay
  Delay3 : xbsIndex_r4/Delay  rst=off  infoeditControl=Selection of Reset will increase slice count due to use of real FFs and instead of SRLs  en=off  latency=1  reg_retiming=off  dbl_ovrd=off  block_type=delay
  Dual Port RAM : xbsIndex_r4/Dual Port RAM  depth=8  initVector=0  distributed_mem=Distributed memory  init_a=0  init_b=0  rst_a=off  rst_b=off  en_a=off  en_b=off  latency=1  write_mode_A=Read After Write  write_mode_B=Read After Write  optimize=Area  dbl_ovrd=off  block_type=dpram
  Register : xbsIndex_r4/Register  init=0  rst=off  en=off  dbl_ovrd=off  block_type=register
  Register1 : xbsIndex_r4/Register  init=0  rst=off  en=off  dbl_ovrd=off  block_type=register
  Relational : xbsIndex_r4/Relational  mode=a=b  op_type=Bool  en=off  latency=1  dbl_ovrd=off  block_type=relational
  Terminator : Terminator
  Terminator1 : Terminator
  IQ out : Outport
  phaseRef out : Outport  Port=2
  wires:
  Constant/1 -> "DDS Compiler 6.0 "/1
  Register1/1 -> Dual Port RAM/2
  Register/1 -> Dual Port RAM/1
  Bus Selector/2 -> Relational/1  "<chan>"
  ID/1 -> Relational/2
  Relational/1 -> Dual Port RAM/3
  Bus Selector/3 -> Register1/1  "<freq>"
  Bus Selector/1 -> Register/1  "<subBand>"
  Delay3/1 -> Delay1/1
  Delay1/1 -> Delay2/1
  Delay2/1 -> "DDS Compiler 6.0 "/3, Bus Creator1/1  "band"
  "DDS Compiler 6.0 "/1 -> Terminator1/1
  Dual Port RAM/1 -> Terminator/1
  Convert/1 -> "DDS Compiler 6.0 "/2, Bus Creator1/2  "DDSphase"
  AddSub/1 -> Convert/1, Delay/1
  band/1 -> Dual Port RAM/4, Delay3/1
  "DDS Compiler 6.0 "/2 -> Bus Creator/1  "Q"
  "DDS Compiler 6.0 "/3 -> Bus Creator/2  "I"
  "DDS Compiler 6.0 "/4 -> Bus Creator/3  "band"
  Bus Creator1/1 -> phaseRef out/1
  Bus Creator/1 -> IQ out/1
  freqBus/1 -> Bus Selector/1
  Dual Port RAM/2 -> AddSub/2
  Delay/1 -> AddSub/1

== system CryoDetLibCMB/demod 8Ch/Set Ampls ==
  note: Set Channel Amplitudes
      | Given its channel ID, scales I&Q by channel amplitude setting
      | interleaved over 8 bands
      | AmplRAM is updated asynchronously to operation
  note: Ampl RAM
  note: Which demodulator channel is this?
  ID : Inport
  amplBus : Inport  Port=2
  DDS IQ : Inport  Port=3
  Bus Creator : BusCreator  Inputs=3
  Bus Selector : BusSelector  OutputSignals=subBand,chan,freq
  Bus Selector1 : BusSelector  OutputSignals=subBand,chan,freq
  Delay1 : xbsIndex_r4/Delay  rst=off  infoeditControl=Selection of Reset will increase slice count due to use of real FFs and instead of SRLs  en=off  latency=1  reg_retiming=off  dbl_ovrd=off  block_type=delay
  Delay2 : xbsIndex_r4/Delay  rst=off  infoeditControl=Selection of Reset will increase slice count due to use of real FFs and instead of SRLs  en=off  latency=3  reg_retiming=off  dbl_ovrd=off  block_type=delay
  Delay4 : xbsIndex_r4/Delay  rst=off  infoeditControl=Selection of Reset will increase slice count due to use of real FFs and instead of SRLs  en=off  latency=1  reg_retiming=off  dbl_ovrd=off  block_type=delay
  Dual Port RAM : xbsIndex_r4/Dual Port RAM  depth=8  initVector=0  distributed_mem=Distributed memory  init_a=0  init_b=0  rst_a=off  rst_b=off  en_a=off  en_b=off  latency=1  write_mode_A=Read After Write  write_mode_B=Read After Write  optimize=Area  dbl_ovrd=off  block_type=dpram
  Mult : xbsIndex_r4/Mult  precision=User Defined  arith_type="Signed  (2's comp)"  n_bits=18  bin_pt=17  quantization=Truncate  overflow=Wrap  en=off  latency=3  use_behavioral_HDL=off  opt=Speed  use_embedded=on  optimum_pipeline=off  pipeline=on  dbl_ovrd=off  use_rpm=on  placement_style=Triangular  block_type=mult
  Mult1 : xbsIndex_r4/Mult  precision=User Defined  arith_type="Signed  (2's comp)"  n_bits=18  bin_pt=17  quantization=Truncate  overflow=Wrap  en=off  latency=3  use_behavioral_HDL=off  opt=Speed  use_embedded=on  optimum_pipeline=off  pipeline=on  dbl_ovrd=off  use_rpm=on  placement_style=Triangular  block_type=mult
  Register : xbsIndex_r4/Register  init=0  rst=off  en=off  dbl_ovrd=off  block_type=register
  Register1 : xbsIndex_r4/Register  init=0  rst=off  en=off  dbl_ovrd=off  block_type=register
  Relational : xbsIndex_r4/Relational  mode=a=b  op_type=Bool  en=off  latency=1  dbl_ovrd=off  block_type=relational
  Terminator : Terminator
  IQ out : Outport
  wires:
  Dual Port RAM/1 -> Terminator/1
  amplBus/1 -> Bus Selector/1
  Register/1 -> Dual Port RAM/1
  Bus Creator/1 -> IQ out/1
  Relational/1 -> Dual Port RAM/3
  Bus Selector/2 -> Relational/1  "<chan>"
  Bus Selector/3 -> Register1/1  "<freq>"
  Bus Selector/1 -> Register/1  "<subBand>"
  Register1/1 -> Dual Port RAM/2
  ID/1 -> Relational/2
  DDS IQ/1 -> Bus Selector1/1
  Bus Selector1/1 -> Dual Port RAM/4, Delay2/1  "<subBand>"
  Bus Selector1/2 -> Delay4/1  "<chan>"
  Bus Selector1/3 -> Delay1/1  "<freq>"
  Delay4/1 -> Mult/2
  Dual Port RAM/2 -> Mult1/1, Mult/1
  Delay1/1 -> Mult1/2
  Mult/1 -> Bus Creator/2
  Mult1/1 -> Bus Creator/3
  Delay2/1 -> Bus Creator/1

== system CryoDetLibCMB/demod 8Ch/phaseRefDownsample ==
  note: Downsample Phase reference and hold the value for each band for 16 ticks so next level interleaver can index across channel
  In1 : Inport
  chanSynch : Inport  Port=2
  BitBasher : xbsIndex_r4/BitBasher  bitexpr=band = {in[7:5]}  display_expr=on  sr_1=band  arith_type1=Unsigned  bin_pt1=0  sr_2=2  arith_type2=Unsigned  bin_pt2=0  sr_3=3  arith_type3=Unsigned  bin_pt3=0  sr_4=4  arith_type4=Unsigned  bin_pt4=0  dbl_ovrd=off  block_type=bitbasher
  Bus Creator : BusCreator  Inputs=2
  Bus Selector : BusSelector  OutputSignals=band,DDSphase
  Constant : xbsIndex_r4/Constant  const=1  gui_display_data_type=Fixed-point  arith_type=Signed (2's comp)  n_bits=7  bin_pt=0  preci_type=Single  exp_width=8  frac_width=24  explicit_period=off  period=1  equ=P=C  opselect=C  inp2=PCIN>>17  opr=+  inp1=P  carry=CIN  dbl_ovrd=off  block_type=constant
  Constant1 : xbsIndex_r4/Constant  const=0  gui_display_data_type=Fixed-point  arith_type=Signed (2's comp)  n_bits=7  bin_pt=0  preci_type=Single  exp_width=8  frac_width=24  explicit_period=off  period=1  equ=P=C  opselect=C  inp2=PCIN>>17  opr=+  inp1=P  carry=CIN  dbl_ovrd=off  block_type=constant
  Convert : xbsIndex_r4/Convert  gui_display_data_type=Boolean  arith_type=Boolean  n_bits=16  bin_pt=14  float_type=Single  exp_bits=8  fraction_bits=24  quantization=Truncate  overflow=Wrap  en=off  latency=0  pipeline=off  dbl_ovrd=off  block_type=convert
  Counter : xbsIndex_r4/Counter  cnt_type=Free Running  cnt_to=Inf  operation=Up  start_count=0  cnt_by_val=1  arith_type=Unsigned  n_bits=7  bin_pt=0  load_pin=on  rst=off  en=off  explicit_period=off  period=1  use_behavioral_HDL=off  implementation=Fabric  dbl_ovrd=off  block_type=counter
  Register : xbsIndex_r4/Register  init=0  rst=off  en=on  dbl_ovrd=off  block_type=register
  Register1 : xbsIndex_r4/Register  init=0  rst=off  en=off  dbl_ovrd=off  block_type=register
  Register2 : xbsIndex_r4/Register  init=0  rst=off  en=on  dbl_ovrd=off  block_type=register
  Register3 : xbsIndex_r4/Register  init=0  rst=off  en=off  dbl_ovrd=off  block_type=register
  Register4 : xbsIndex_r4/Register  init=0  rst=off  en=off  dbl_ovrd=off  block_type=register
  Relational : xbsIndex_r4/Relational  mode=a=b  op_type=Bool  en=off  latency=1  dbl_ovrd=off  block_type=relational
  Relational1 : xbsIndex_r4/Relational  mode=a=b  op_type=Bool  en=off  latency=1  dbl_ovrd=off  block_type=relational
  Out1 : Outport
  wires:
  In1/1 -> Bus Selector/1
  chanSynch/1 -> Convert/1
  Constant/1 -> Counter/2
  Convert/1 -> Counter/1
  Counter/1 -> Relational1/1, BitBasher/1
  BitBasher/1 -> Register3/1, Relational/2
  Bus Selector/1 -> Relational/1  "<band>"
  Relational/1 -> Register/2
  Bus Selector/2 -> Register1/1  "<DDSphase>"
  Register1/1 -> Register/1
  Constant1/1 -> Relational1/2
  Register/1 -> Register2/1
  Relational1/1 -> Register2/2
  Register2/1 -> Bus Creator/2
  Bus Creator/1 -> Out1/1
  Register3/1 -> Register4/1
  Register4/1 -> Bus Creator/1

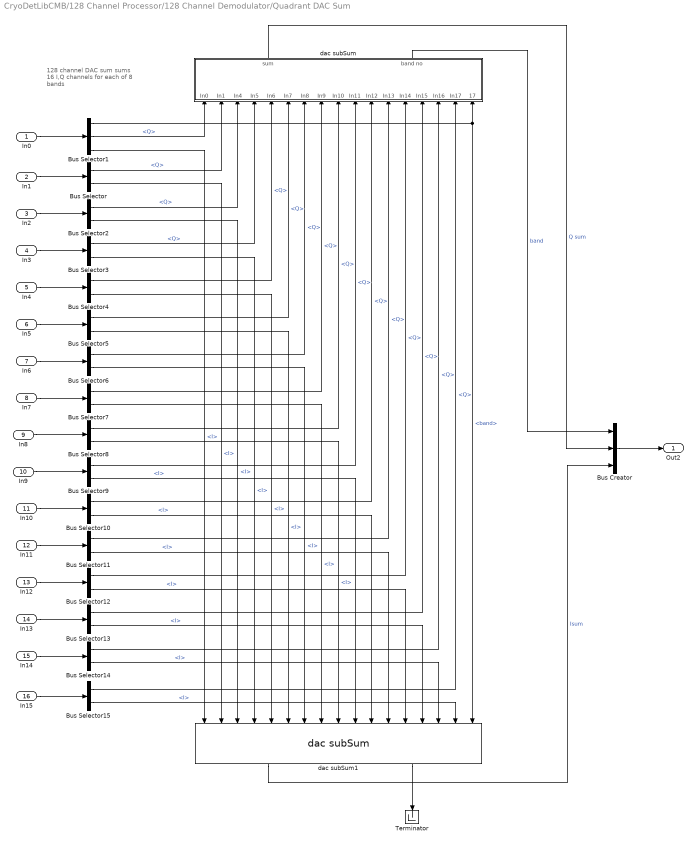
== system CryoDetLibCMB/128 Channel Processor/128 Channel Demodulator/Quadrant DAC Sum ==
  note: 128 channel DAC sum
      | sums 16 I,Q channels for each of 8 bands
  In0 : Inport
  In1 : Inport  Port=2
  In2 : Inport  Port=3
  In3 : Inport  Port=4
  In4 : Inport  Port=5
  In5 : Inport  Port=6
  In6 : Inport  Port=7
  In7 : Inport  Port=8
  In8 : Inport  Port=9
  In9 : Inport  Port=10
  In10 : Inport  Port=11
  In11 : Inport  Port=12
  In12 : Inport  Port=13
  In13 : Inport  Port=14
  In14 : Inport  Port=15
  In15 : Inport  Port=16
  Bus Creator : BusCreator  Inputs=3
  Bus Selector{,2..15} (15 alike) : BusSelector  OutputSignals=Q,I
  Bus Selector1 : BusSelector  OutputSignals=band,Q,I
  Terminator : Terminator
  dac subSum : Subsystem
  dac subSum1 : CryoDetLibCMB/128 Channel Processor/128 Channel Demodulator/Quadrant DAC Sum/dac subSum
  Out2 : Outport
  wires:
  In1/1 -> Bus Selector/1
  In0/1 -> Bus Selector1/1
  In2/1 -> Bus Selector2/1
  In3/1 -> Bus Selector3/1
  In4/1 -> Bus Selector4/1
  In5/1 -> Bus Selector5/1
  In6/1 -> Bus Selector6/1
  In7/1 -> Bus Selector7/1
  In8/1 -> Bus Selector8/1
  In9/1 -> Bus Selector9/1
  In10/1 -> Bus Selector10/1
  In11/1 -> Bus Selector11/1
  In12/1 -> Bus Selector12/1
  In13/1 -> Bus Selector13/1
  In14/1 -> Bus Selector14/1
  In15/1 -> Bus Selector15/1
  Bus Selector1/2 -> dac subSum/1(In0)  "<Q>"
  Bus Selector/1 -> dac subSum/2(In1)  "<Q>"
  Bus Selector2/1 -> dac subSum/3(In4)  "<Q>"
  Bus Selector3/1 -> dac subSum/4(In5)  "<Q>"
  Bus Selector4/1 -> dac subSum/5(In6)  "<Q>"
  Bus Selector5/1 -> dac subSum/6(In7)  "<Q>"
  Bus Selector6/1 -> dac subSum/7(In8)  "<Q>"
  Bus Selector7/1 -> dac subSum/8(In9)  "<Q>"
  Bus Selector8/1 -> dac subSum/9(In10)  "<Q>"
  Bus Selector9/1 -> dac subSum/10(In11)  "<Q>"
  Bus Selector10/1 -> dac subSum/11(In12)  "<Q>"
  Bus Selector11/1 -> dac subSum/12(In13)  "<Q>"
  Bus Selector12/1 -> dac subSum/13(In14)  "<Q>"
  Bus Selector13/1 -> dac subSum/14(In15)  "<Q>"
  Bus Selector14/1 -> dac subSum/15(In16)  "<Q>"
  Bus Selector15/1 -> dac subSum/16(In17)  "<Q>"
  Bus Selector1/1 -> dac subSum/17(band in), dac subSum1/17  "<band>"
  Bus Selector15/2 -> dac subSum1/16  "<I>"
  Bus Selector14/2 -> dac subSum1/15  "<I>"
  Bus Selector13/2 -> dac subSum1/14  "<I>"
  Bus Selector12/2 -> dac subSum1/13  "<I>"
  Bus Selector11/2 -> dac subSum1/12  "<I>"
  Bus Selector10/2 -> dac subSum1/11  "<I>"
  Bus Selector9/2 -> dac subSum1/10  "<I>"
  Bus Selector8/2 -> dac subSum1/9  "<I>"
  Bus Selector7/2 -> dac subSum1/8  "<I>"
  Bus Selector6/2 -> dac subSum1/7  "<I>"
  Bus Selector5/2 -> dac subSum1/6  "<I>"
  Bus Selector4/2 -> dac subSum1/5  "<I>"
  Bus Selector3/2 -> dac subSum1/4  "<I>"
  Bus Selector2/2 -> dac subSum1/3  "<I>"
  Bus Selector/2 -> dac subSum1/2  "<I>"
  Bus Selector1/3 -> dac subSum1/1  "<I>"
  Bus Creator/1 -> Out2/1
  dac subSum/2(band no) -> Bus Creator/1  "band"
  dac subSum/1(sum) -> Bus Creator/2  "Q sum"
  dac subSum1/1 -> Bus Creator/3  "Isum"
  dac subSum1/2 -> Terminator/1

== system CryoDetLibCMB/128 Channel Processor/Loop Filter/initial Frequencies1 ==
  note: initial Frequencies
  note: select initial frequency
      | for now just mux from input registers
      | eventually configure RAM and loading protocol
  channel : Inport
  Gateway Out12 : xbsIndex_r4/Gateway Out  inherit_from_input=off  hdl_port=off  rows=1  columns=1  UseAsDAC=off  DACChannel='1'  interface=None  automatic_assignment=on  address_offset=hex2dec('00')  intf_name=''  intf_description=''  timing_constraint=None  locs_specified=off  LOCs={}  io_standard={}  block_type=gatewayout
  Gateway Out13 : xbsIndex_r4/Gateway Out  inherit_from_input=off  hdl_port=off  rows=1  columns=1  UseAsDAC=off  DACChannel='1'  interface=None  automatic_assignment=on  address_offset=hex2dec('00')  intf_name=''  intf_description=''  timing_constraint=None  locs_specified=off  LOCs={}  io_standard={}  block_type=gatewayout
  Mux : xbsIndex_r4/Mux  inputs=16  en=off  latency=1  precision=Full  arith_type=Unsigned  n_bits=24  bin_pt=24  quantization=Truncate  overflow=Wrap  dbl_ovrd=off  block_type=mux
  initial Freqs : Scope  NumInputPorts=2
  Fi : Outport
  wires:
  channel/1 -> Gateway Out12/1, Mux/1
  [F0] -> Mux/2
  [F1] -> Mux/3
  [F2] -> Mux/4
  [F3] -> Mux/5
  [F4] -> Mux/6
  [F5] -> Mux/7
  [F6] -> Mux/8
  [F7] -> Mux/9
  [F8] -> Mux/10
  [F9] -> Mux/11
  [F10] -> Mux/12
  [F11] -> Mux/13
  Mux/1 -> Gateway Out13/1, Fi/1
  Gateway Out13/1 -> initial Freqs/2
  Gateway Out12/1 -> initial Freqs/1
  [F15] -> Mux/17
  [F13] -> Mux/15
  [F12] -> Mux/14
  [F14] -> Mux/16
